simulink model "systemAnalysis"  (R2020a)
settings: Solver=VariableStepAuto  StartTime=0.0  StopTime=10.0  MaxStep=0.001  RelTol=1e-3
values from neighbouring files (symbols this model uses):
  g = 9.8    [code.m]    (also in main.m)
  m = 0.11    [code.m]    (also in main.m)
  x_0 = [0.4 0.2 deg2rad(1) deg2rad(0.3)]    [code.m]    (also in main.m)
libraries: helperLibrary x1
settings Model: Creator=danth  LastModifiedBy=danth

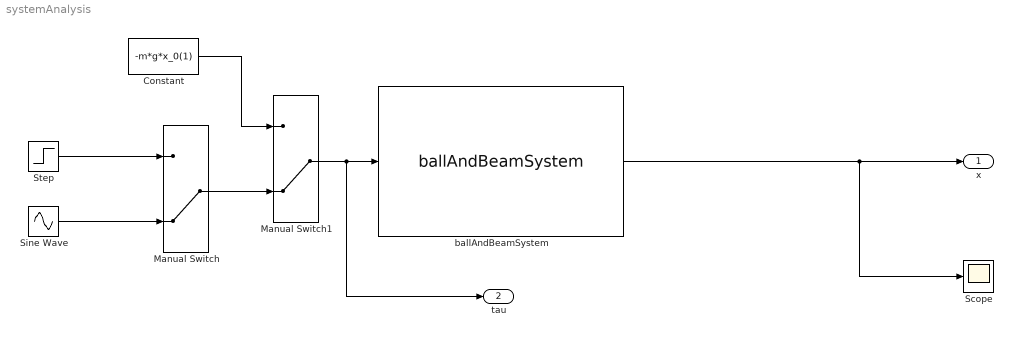
== system systemAnalysis ==
  Constant : Constant  Value=-m*g*x_0(1)
  Manual Switch : ManualSwitch  CurrentSetting=0
  Manual Switch1 : ManualSwitch  CurrentSetting=0
  Scope : Scope
  Sine Wave : Sin  Amplitude=0.2  Frequency=100*2*pi  Phase=pi/2  SampleTime=0
  Step : Step  Time=0.1  After=0.1  SampleTime=0
  ballAndBeamSystem : helperLibrary/ballAndBeamSystem  SystemSampleTime=-1  Latency=0  AutoFrameSizeCalculation=off
  x : Outport
  tau : Outport  Port=2
  wires:
  ballAndBeamSystem/1 -> x/1, Scope/1
  Step/1 -> Manual Switch/1
  Sine Wave/1 -> Manual Switch/2
  Manual Switch1/1 -> tau/1, ballAndBeamSystem/1
  Manual Switch/1 -> Manual Switch1/2
  Constant/1 -> Manual Switch1/1
